simulink model "Hector"  (R2023b)
settings: Solver=daessc  StartTime=0.0  StopTime=1  FixedStep=0.001  MaxStep=1e-3  RelTol=1e-2
model workspace (MATLAB code in the model file):
  | %% World Plane
  | plane_x = 20;
  | plane_y = 2;
  | plane_z = 0.05;
  | 
  | %% motor
  | %A1
  | motor_com = [0, -0.02,0];
  | motor_com_mirror = [0, 0.02,0];
  | 
  | motor_I = [0.00048,0.00071,0.00048];
  | motor_mass = 0.605;
  | 
  | %% Body
  | % Inertial
  | body_com_x = 0.0;
  | body_com_y = 0.0;
  | body_com_z = -0.0;
  | body_mass = 5.75;
  | body_ixx = 44350*1e-6;
  | body_ixy = 0.0;
  | body_ixz = 0.0;
  | body_iyy = 53149*1e-6;
  | body_iyz = 0.0;
  | body_izz = 21390*1e-6;
  | 
  | %% Hip 1
  | % joint
  | hip1_offset_x =0.0;
  | hip1_offset_y = 0.047;
  | hip1_offset_z = 0.1265;
  | % hip1_max = 15;
  | % hip1_min = -15;
  | hip1_velocity_max = 21;
  | hip1_torque_max = 33.5;
  | % Inertial
  | hip1_com_x = 0.0268;
  | hip1_com_y = -0.00315;
  | hip1_com_z = -0.0272;
  | hip1_mass = 0.173;
  | hip1_ixx = 0.00022;
  | hip1_ixy = 0.0;
  | hip1_ixz = 0.0;
  | hip1_iyy = 0.00024;
  | hip1_iyz = 0.0;
  | hip1_izz = 0.00016;
  | 
  | %% Hip 2
  | % joint
  | hip2_offset_x =0.053;
  | hip2_offset_y = 0.0185;
  | hip2_offset_z = 0.071;
  | % hip2_max = 15;
  | % hip2_min = -15;
  | hip2_velocity_max = 21;
  | hip2_torque_max = 33.5;
  | % Inertial
  | hip2_com_x = -0.0308;
  | hip2_com_y = -0.00942;
  | hip2_com_z = 0.0;
  | hip2_mass = 0.0722;
  | hip2_ixx = 0.0000422;
  | hip2_ixy = 0.0;
  | hip2_ixz = 0.0;
  | hip2_iyy = 0.000120;
  | hip2_iyz = 0.0;
  | hip2_izz = 0.0000708;
  | 
  | %% Thigh
  | % joint
  | thigh_offset_x =-0.06;
  | thigh_offset_y = 0.004;
  | thigh_offset_z = 0.0;
  | % thigh_max = 130;
  | % thigh_min = -45;
  | thigh_velocity_max = 21;
  | thigh_torque_max = 33.5;
  | % Inertial
  | thigh_com_x = -0.00143;
  | thigh_com_y = -0.02106;
  | thigh_com_z = -0.06115;
  | thigh_mass = 0.397;
  | thigh_ixx = 0.00197;
  | thigh_ixy = 0.0;
  | thigh_ixz = 0.0;
  | thigh_iyy = 0.00218;
  | thigh_iyz = 0.0;
  | thigh_izz = 0.00033;
  | 
  | ankle_motor_offset_x = 0;
  | ankle_motor_offset_y = 0.039;
  | ankle_motor_offset_z = 0;
  | 
  | knee_motor_offset_x = 0;
  | knee_motor_offset_y = 0.039;
  | knee_motor_offset_z = -0.095;
  | 
  | %% Calf
  | % joint
  | calf_offset_x = 0.0;
  | calf_offset_y = 0.003;
  | calf_offset_z = -0.22;
  | % calf_max = 0;
  | % calf_min = -135;
  | % knee_max = 0;
  | % knee_min = -160;
  | calf_velocity_max = 14*1.5;
  | calf_torque_max = 51;
  | % Inertial
  | calf_com_x = 0.00165;
  | calf_com_y = -0.01117;
  | calf_com_z = -0.06438;
  | calf_mass = 0.136;
  | calf_ixx = 0.00071;
  | calf_ixy = 0.0;
  | calf_ixz = 0.0;
  | calf_iyy = 0.00072;
  | calf_iyz = 0.0;
  | calf_izz = 0.00002;
  | 
  | %% Toe
  | % joint
  | toe_offset_x = 0.0;
  | toe_offset_y = 0.011;
  | toe_offset_z = -0.22;
  | % toe_max = 60;
  | % toe_min = -60;
  | toe_velocity_max = 21;
  | toe_torque_max = 33.5;
  | % Inertial
  | toe_com_x = 0.00239;
  | toe_com_y = 0.00002;
  | toe_com_z = -0.02261;
  | toe_mass = 0.08425;
  | toe_ixx = 0.00001;
  | toe_ixy = 0.0;
  | toe_ixz = 0.0;
  | toe_iyy = 0.00011;
  | toe_iyz = 0.0;
  | toe_izz = 0.00011;
  | %% Contact
  | contact_front = 0.091;
  | contact_rear = -0.061;
  | contact_right = 0.026;
  | contact_left = 0.01;
  | contact_z = 0.039;
  | 
  | %%
  | %dorito
  | dorito_offset_x = 0;
  | dorito_offset_y = 0.012;
  | dorito_offset_z = 0;
  | 
  | dorito_lower_connection = [0.034 0 -0.044];
  | dorito_upper_connection = [0.034 0 0.021];
  | 
  | linkage_mass = 0.051;
  | linkage_com = [0 0 -0.11];
  | linkage_I = [0.00001 0.00002 0.00002];
  | %% Arms
  | shoulder_com_x = 0;
  | shoulder_com_y = 0;
  | shoulder_com_z = 0;
  | shoulder_mass = 0.835;
  | % shoulder_mass = 0.05;
  | shoulder_ixx = 920*1e-6;
  | shoulder_ixy = 0.0;
  | shoulder_ixz = 0.0;
  | shoulder_iyy = 270*1e-6;
  | shoulder_iyz = 0.0;
  | shoulder_izz = 499*1e-6;
  | 
  | upperarm_com_x = 0;
  | upperarm_com_y = 0;
  | upperarm_com_z = 0;
  | upperarm_mass = 1.35;
  | % upperarm_mass = 0.05;
  | upperarm_ixx = 1200*1e-6;
  | upperarm_ixy = 0.0;
  | upperarm_ixz = 0.0;
  | upperarm_iyy = 1170*1e-6;
  | upperarm_iyz = 0.0;
  | upperarm_izz = 729*1e-6;
  | 
  | forearm_com_x = 0;
  | forearm_com_y = 0;
  | forearm_com_z = -0.10;
  | forearm_mass = 0.53;
  | % forearm_mass = 0.03;
  | forearm_ixx = 427*1e-6;
  | forearm_ixy = 0.0;
  | forearm_ixz = 0.0;
  | forearm_iyy = 466*1e-6;
  | forearm_iyz = 0.0;
  | forearm_izz = 72*1e-6;
values from neighbouring files (symbols this model uses):
  body_v0 = [0 0 0]    [Initiate_Simulation.m]
  body_z0 = 0.55    [Initiate_Simulation.m]
  dt_MPC = gaitcycle/10    (= 0.04)    [Initiate_Simulation.m]
  N = 5000    [Initiate_Simulation.m]
  shoulderx_max = 90    [Initiate_Simulation.m]
  shoulderx_min = -15    [Initiate_Simulation.m]
  shoulderx_q0 = 0    [Initiate_Simulation.m]
undefined symbols (not defined in the file or in its folder): AssignMPCStage, sigbuilder_block, X, Y, Z
libraries: sm_lib x169, nesl_utility x95, dspindex x1, simulink x1
(part 1 of 7)
settings Model: Creator=alber  LastModifiedBy=chuon
settings SolverCC: DaesscMode=Balanced  ShapePreserveControl=EnableAll  ZeroCrossAlgorithm=Adaptive  AlgebraicLoopSolver=TrustRegion
settings DataIOCC: LimitDataPoints=on  MaxDataPoints=10000
settings OptimizationCC: LifeSpan=inf
settings DebuggingCC: IgnoredZcDiagnostic=none  UnconnectedInputMsg=warning  UnconnectedOutputMsg=warning  UnconnectedLineMsg=warning  AllowSymbolicDim=off  SFUnexpectedBacktrackingDiag=warning  SFNoUnconditionalDefaultTransitionDiag=warning  SFExecutionAtInitializationDiag=none  ArithmeticOperatorsInVariantConditions=warning
settings ModelReferenceCC: EnableRefExpFcnMdlSchedulingChecks=on
settings SFSimCC: SimUseLocalCustomCode=off  CustomCodeUndefinedFunction=UseInterfaceOnly
settings RTWCC: RTWUseLocalCustomCode=off  DLArmComputeVersion=19.05
settings CodeAppCC: StateflowObjectComments=on
settings GRTTargetCC: TargetLangStandard=C89/C90 (ANSI)
settings ConfigComp: CovMetricSettings=dw  CovSaveCumulativeToWorkspaceVar=on  CovSaveSingleToWorkspaceVar=on  CovExternalEMLEnable=off  CovSFcnEnable=off
settings SimscapeCC: SimscapeLogType=all  SimscapeLogSimulationStatistics=on  SimscapeLogDataHistory=10000
settings ExplorerConfigSet: InternalSimMechanicsExplorerSettings="<ExplorerConfiguration><canonicalview>default</canonicalview><AnimationSetting><BasePlaybackSpeed>1.0</BasePlaybackSpeed><PlaybackSpeedFactor>1.0</PlaybackSpeedFactor></AnimationSetting><TilePanel><TileInfo><Tiles Columns=\"1\" Count=\"1\" Rows=\"1\"><Column Weight=\"1\"/><Row Weight=\"1\"/><Tile Height=\"1\" Width=\"1\" X=\"0\" Y=\"0\"/></Tiles></TileInfo><SceneInfo><SceneViewer><BGColor><R>0.60000002384185791</R><G>0.60000002384185791</G><B>0.60000002384185791</B></BGColor><Camera><DoPerspective>off</DoPerspective><Position><X>4.09836314786391398</X><Y>-3.96594002614336105</Y><Z>4.23361424387727237</Z></Position><Center><X>-0.00094258239399230663</X><Y>0.133365704114546013</Y><Z>0.134308513619366465</Z></Center><Up><X>-0.408248290463863073</X><Y>0.408248290463863073</Y><Z>0.816496580927726145</Z></Up><ViewLimDist>1</ViewLimDist><YLim>0.846160332563345552</YLim><XLim>1.21706171949998887</XLim></Camera></SceneViewer></SceneInfo></TilePanel><MechEditorPanel><Cameras/><GfxPanelCameraMap/><VideoCreator><PlaybackSpeedRatio>1.0</PlaybackSpeedRatio><FrameRate>60</FrameRate><VideoFormat>Motion JPEG AVI</VideoFormat><FrameSize>[800 600]</FrameSize></VideoCreator></MechEditorPanel></ExplorerConfiguration>"

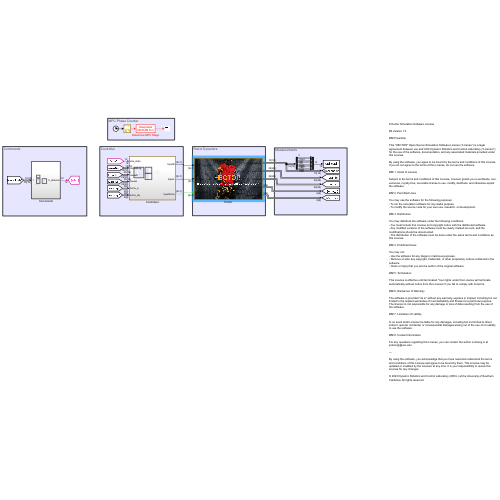
[thumbnail: Simulink's stored preview of the top-level diagram]
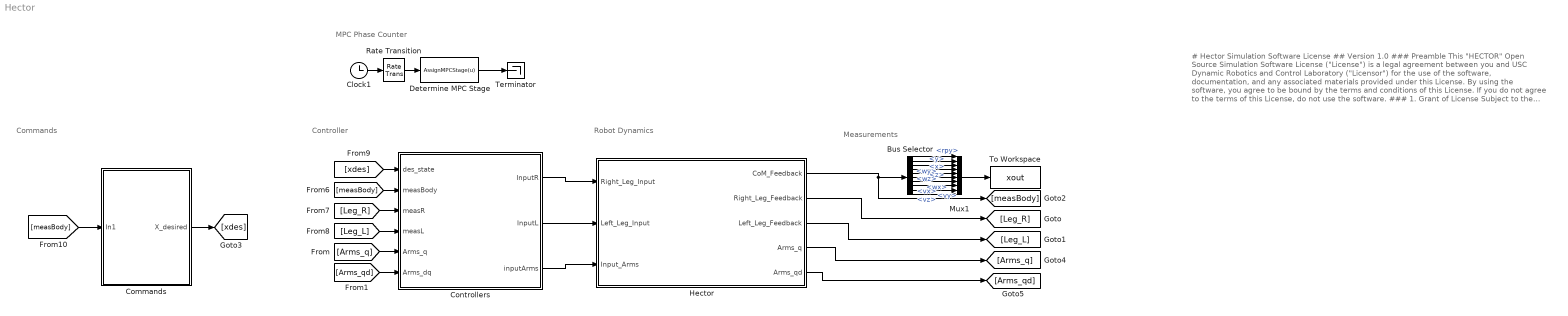
== system Hector ==
  note: # Hector Simulation Software License
      |
      | ## Version 1.0
      |
      | ### Preamble
      |
      | This "HECTOR" Open Source Simulation Software License ("License") is a legal agreement between you and USC Dynamic Robotics and Control Laboratory ("Licensor") for the use of the software, documentation, and any associated materials provided under this License.
      |
      | By using the software, you agree to be bound by the terms and conditions of this License. If you do not agree to the terms of this License, do not use the software.
      |
      | ### 1. Grant of License
      |
      | Subject to the terms and conditions of this License, Licensor grants you a worldwide, non-exclusive, royalty-free, revocable license to use, modify, distribute, and otherwise exploit the software.
      |
      | ### 2. Permitted Uses
      |
      | You may use the software for the following purposes:
      | - To run the simulation software for any lawful purpose.
      | - To modify the source code for your own use, research, or development.
      |
      | ### 3. Distribution
      |
      | You may distribute the software under the following conditions:
      | - You must include this License and copyright notice with the distributed software.
      | - Any modified versions of the software must be clearly marked as such, and the modifications should be documented.
      | - The distribution of the software must be done under the same terms and conditions as this License.
      |
      | ### 4. Prohibited Uses
      |
      | You may not:
      | - Use the software for any illegal or malicious purposes.
      | - Remove or alter any copyright, trademark, or other proprietary notices contained in the software.
      | - Claim or imply that you are the author of the original software.
      |
      | ### 5. Termination
      |
      | This License is effective until terminated. Your rights under this License will terminate automatically without notice from the Licensor if you fail to comply with its terms.
      |
      | ### 6. Disclaimer of Warranty
      |
      | The software is provided "as is" without any warranty, express or implied, including but not limited to the implied warranties of merchantability and fitness for a particular purpose. The licensor is not responsible for any damage or loss of data resulting from the use of the software.
      |
      | ### 7. Limitation of Liability
      |
      | In no event shall Licensor be liable for any damages, including but not limited to direct, indirect, special, incidental, or consequential damages arising out of the use of or inability to use the software.
      |
      | ### 8. Contact Information
      |
      | For any questions regarding this License, you can contact the author Junheng Li at junhengl@usc.edu.
      |
      | ---
      |
      | By using the software, you acknowledge that you have read and understood the terms and conditions of this License and agree to be bound by them. This License may be updated or modified by the Licensor at any time. It is your responsibility to review this License for any changes.
      |
      | © 2023 Dynamic Robotics and Control Laboratory (DRCL) at the University of Southern California. All rights reserved.
  note: Measurements
  note: MPC Phase Counter
  note: Commands
  note: Robot Dynamics
  note: Controller
  Bus Selector : BusSelector  OutputSignals=rpy,x,y,z,wz,wy,wx,vx,vy,vz
  Clock1 : Clock
  Commands : Subsystem
  Controllers : Subsystem
  Determine MPC Stage : MATLABFcn  MATLABFcn=AssignMPCStage(u)  Output1D=off
  Hector : Subsystem
      mask Display: image('$imagefile'); % Use "Edit Image" on toolstrip to change.
  Mux1 : Mux  Inputs=10
  Rate Transition : RateTransition  OutPortSampleTime=5e-4
  Terminator : Terminator
  To Workspace : ToWorkspace  VariableName=xout  SampleTime=-1
  wires:
  Hector/2(Right_Leg_Feedback) -> [Leg_R]
  Hector/3(Left_Leg_Feedback) -> [Leg_L]
  Hector/1(CoM_Feedback) -> [measBody], Bus Selector/1
  [Leg_L] -> Controllers/4(measL)
  [Leg_R] -> Controllers/3(measR)
  [measBody] -> Controllers/2(measBody)
  Controllers/1(InputR) -> Hector/1(Right_Leg_Input)
  Controllers/2(InputL) -> Hector/2(Left_Leg_Input)
  Bus Selector/1 -> Mux1/1  "<rpy>"
  Bus Selector/2 -> Mux1/2  "<x>"
  Bus Selector/3 -> Mux1/3  "<y>"
  Bus Selector/4 -> Mux1/4  "<z>"
  Bus Selector/5 -> Mux1/5  "<wz>"
  Bus Selector/7 -> Mux1/7  "<wx>"
  Bus Selector/8 -> Mux1/8  "<vx>"
  Bus Selector/9 -> Mux1/9  "<vy>"
  Bus Selector/10 -> Mux1/10  "<vz>"
  Bus Selector/6 -> Mux1/6  "<wy>"
  Mux1/1 -> To Workspace/1
  [xdes] -> Controllers/1(des_state)
  Clock1/1 -> Rate Transition/1
  Rate Transition/1 -> Determine MPC Stage/1
  [measBody] -> Commands/1(In1)
  Commands/1(X_desired) -> [xdes]
  Determine MPC Stage/1 -> Terminator/1
  Hector/4(Arms_q) -> [Arms_q]
  Hector/5(Arms_qd) -> [Arms_qd]
  Controllers/3(inputArms) -> Hector/3(Input_Arms)
  [Arms_q] -> Controllers/5(Arms_q)
  [Arms_qd] -> Controllers/6(Arms_dq)

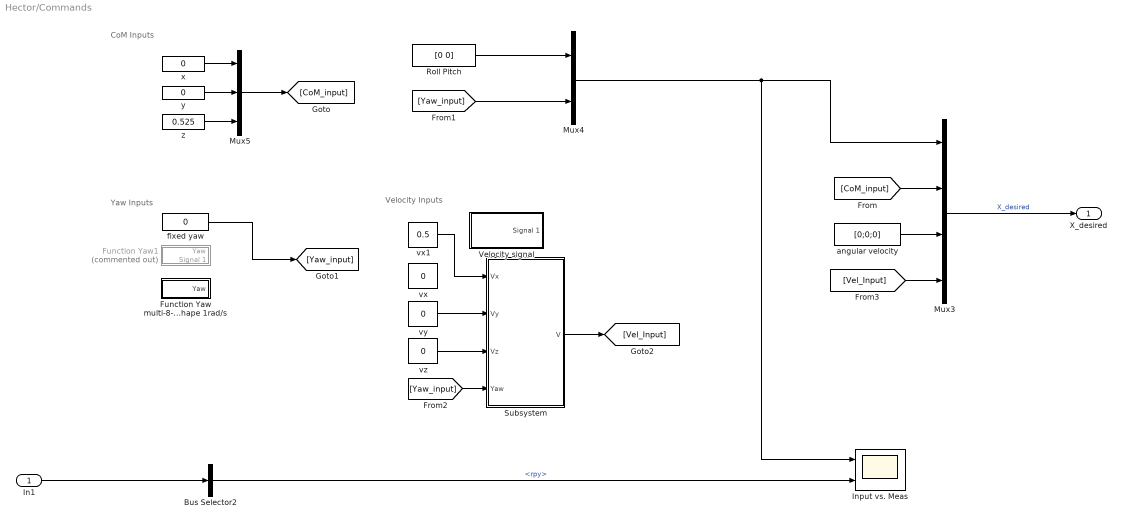
== system Hector/Commands ==
  note: Velocity Inputs
  note: CoM Inputs
  note: Yaw Inputs
  In1 : Inport
  Bus Selector2 : BusSelector  OutputSignals=rpy
  Function Yaw multi-8-shape 1rad/s : Subsystem  Tag=STV Subsys  LoadFcn=sigbuilder_block('load');  StartFcn=sigbuilder_block('start');  StopFcn=sigbuilder_block('stop');  ClipboardFcn=sigbuilder_block('clipboard');  mask(Sigbuilder block){tuvar=[0:10]}
      mask help: Simulink:masks:SigbuilderBlock_MD
      mask init:
      | if ~strcmp(get_param(bdroot(gcbh),'SimulationStatus'),'stopped') tuvar = sigbuilder_block('maskInit'); end
      settings: CopyFcn=sigbuilder_block('copy');  DeleteFcn=sigbuilder_block('delete');  ModelCloseFcn=sigbuilder_block('modelClose');  PreSaveFcn=sigbuilder_block('preSave');  PauseFcn=sigbuilder_block('pause');  ContinueFcn=sigbuilder_block('continue');  NameChangeFcn=sigbuilder_block('namechange');  OpenFcn=sigbuilder_block('open',[595.8 225 550.8 361.2 ]);  CloseFcn=sigbuilder_block('close');
      mask Display: plot(0, 0, 100, 100,[2, 2, 32, 32, 2], [68, 8, 8, 68, 68],[32, 2], [38, 38], [32, 19, 2],[53, 60, 44], [32, 17, 17, 2],[16, 16, 31, 31]);txt = getActiveGroup(gcbh);text(2, 100, txt,'verticalAlignment', 'top');
  Function Yaw1 : Subsystem  Tag=STV Subsys  Commented=on  LoadFcn=sigbuilder_block('load');  StartFcn=sigbuilder_block('start');  StopFcn=sigbuilder_block('stop');  ClipboardFcn=sigbuilder_block('clipboard');  mask(Sigbuilder block){tuvar=[0:10]}
      mask help: Simulink:masks:SigbuilderBlock_MD
      mask init:
      | if ~strcmp(get_param(bdroot(gcbh),'SimulationStatus'),'stopped') tuvar = sigbuilder_block('maskInit'); end
      settings: CopyFcn=sigbuilder_block('copy');  DeleteFcn=sigbuilder_block('delete');  ModelCloseFcn=sigbuilder_block('modelClose');  PreSaveFcn=sigbuilder_block('preSave');  PauseFcn=sigbuilder_block('pause');  ContinueFcn=sigbuilder_block('continue');  NameChangeFcn=sigbuilder_block('namechange');  OpenFcn=sigbuilder_block('open',[190.2 83.4 493.2 502.8 ]);  CloseFcn=sigbuilder_block('close');
      mask Display: plot(0, 0, 100, 100,[2, 2, 32, 32, 2], [68, 8, 8, 68, 68],[32, 2], [38, 38], [32, 19, 2],[53, 60, 44], [32, 17, 17, 2],[16, 16, 31, 31]);txt = getActiveGroup(gcbh);text(2, 100, txt,'verticalAlignment', 'top');
  Input vs. Meas : Scope  NumInputPorts=2
  Mux3 : Mux
  Mux4 : Mux  Inputs=2
  Mux5 : Mux  Inputs=3
  Roll Pitch : Constant  Value=[0 0]
  Subsystem : Subsystem
  Velocity signal : Subsystem  Tag=STV Subsys  LoadFcn=sigbuilder_block('load');  StartFcn=sigbuilder_block('start');  StopFcn=sigbuilder_block('stop');  ClipboardFcn=sigbuilder_block('clipboard');  mask(Sigbuilder block){tuvar=[0:10]}
      mask help: Simulink:masks:SigbuilderBlock_MD
      mask init:
      | if ~strcmp(get_param(bdroot(gcbh),'SimulationStatus'),'stopped') tuvar = sigbuilder_block('maskInit'); end
      settings: CopyFcn=sigbuilder_block('copy');  DeleteFcn=sigbuilder_block('delete');  ModelCloseFcn=sigbuilder_block('modelClose');  PreSaveFcn=sigbuilder_block('preSave');  PauseFcn=sigbuilder_block('pause');  ContinueFcn=sigbuilder_block('continue');  NameChangeFcn=sigbuilder_block('namechange');  OpenFcn=sigbuilder_block('open',[439.8 157.8 550.8 400.2 ]);  CloseFcn=sigbuilder_block('close');
      mask Display: plot(0, 0, 100, 100,[2, 2, 32, 32, 2], [68, 8, 8, 68, 68],[32, 2], [38, 38], [32, 19, 2],[53, 60, 44], [32, 17, 17, 2],[16, 16, 31, 31]);txt = getActiveGroup(gcbh);text(2, 100, txt,'verticalAlignment', 'top');
  angular velocity : Constant  Value=[0;0;0]
  fixed yaw : Constant  Value=0
  vx : Constant  Value=0
  vx1 : Constant  Value=0.5
  vy : Constant  Value=0
  vz : Constant  Value=0
  x : Constant  Value=0
  y : Constant  Value=0
  z : Constant  Value=0.525
  X_desired : Outport
  wires:
  y/1 -> Mux5/2
  Mux4/1 -> Mux3/1, Input vs. Meas/1
  x/1 -> Mux5/1
  angular velocity/1 -> Mux3/3
  Roll Pitch/1 -> Mux4/1
  z/1 -> Mux5/3
  In1/1 -> Bus Selector2/1
  Bus Selector2/1 -> Input vs. Meas/2  "<rpy>"
  Mux3/1 -> X_desired/1  "X_desired"
  Mux5/1 -> [CoM_input]
  [CoM_input] -> Mux3/2
  vx1/1 -> Subsystem/1(Vx)
  vy/1 -> Subsystem/2(Vy)
  vz/1 -> Subsystem/3(Vz)
  fixed yaw/1 -> [Yaw_input]
  [Yaw_input] -> Mux4/2
  [Yaw_input] -> Subsystem/4(Yaw)
  Subsystem/1(V) -> [Vel_Input]
  [Vel_Input] -> Mux3/4

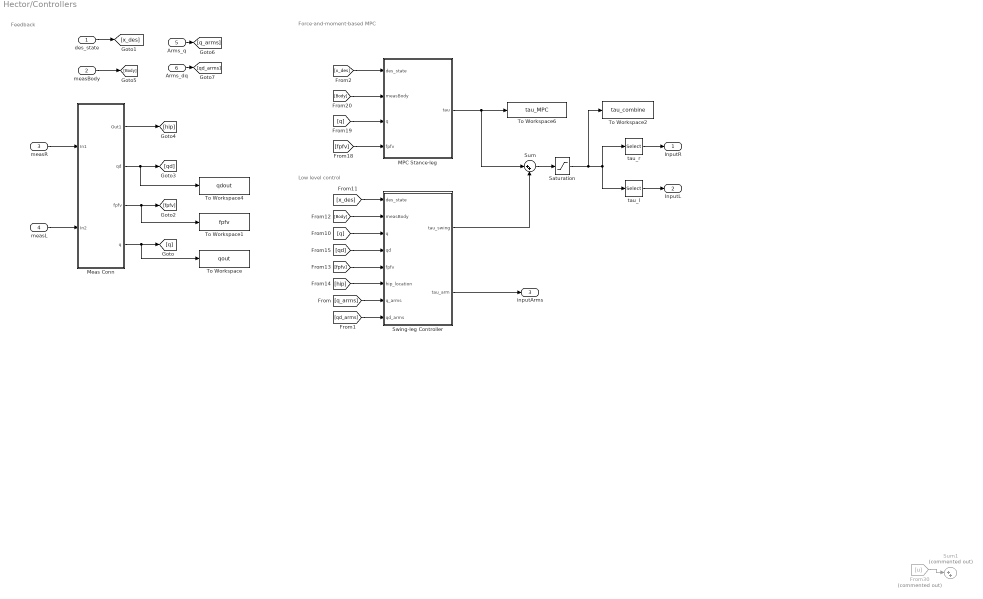
== system Hector/Controllers ==
  note: Low level control
  note: Force-and-moment-based MPC
  note: Feedback
  des_state : Inport
  measBody : Inport  Port=2
  measR : Inport  Port=3
  measL : Inport  Port=4
  Arms_q : Inport  Port=5
  Arms_dq : Inport  Port=6
  From30 : From  Commented=on  GotoTag=u
  MPC Stance-leg : Subsystem  TreatAsAtomicUnit=on
  Meas Conn : Subsystem
  Saturation : Saturate  UpperLimit=[33.5;33.5;33.5;51;33.5;33.5;33.5;33.5;51;33.5]*1  LowerLimit=-[33.5;33.5;33.5;51;33.5;33.5;33.5;33.5;51;33.5]*1
  Sum : Sum  Inputs=|++
  Sum1 : Sum  Commented=on  Inputs=|++
  "Swing-leg Controller " : Subsystem
  To Workspace : ToWorkspace  VariableName=qout  SampleTime=-1
  To Workspace1 : ToWorkspace  VariableName=fpfv  SampleTime=-1
  To Workspace2 : ToWorkspace  VariableName=tau_combine  SampleTime=-1
  To Workspace4 : ToWorkspace  VariableName=qdout  SampleTime=-1
  To Workspace6 : ToWorkspace  VariableName=tau_MPC  SampleTime=-1
  tau_l : Selector  InputPortWidth=10  IndexOptions=Index vector (dialog)  Indices=[6:10]  OutputSizes=1
  tau_r : Selector  InputPortWidth=10  IndexOptions=Index vector (dialog)  Indices=[1:5]  OutputSizes=1
  InputR : Outport
  InputL : Outport  Port=2
  inputArms : Outport  Port=3
  wires:
  measBody/1 -> [Body]
  tau_r/1 -> InputR/1
  tau_l/1 -> InputL/1
  Saturation/1 -> To Workspace2/1, tau_l/1, tau_r/1
  Sum/1 -> Saturation/1
  des_state/1 -> [x_des]
  [x_des] -> MPC Stance-leg/1(des_state)
  [x_des] -> "Swing-leg Controller "/1(des_state)
  [Body] -> "Swing-leg Controller "/2(measBody)
  [q] -> "Swing-leg Controller "/3(q)
  [fpfv] -> "Swing-leg Controller "/5(fpfv)
  [hip] -> "Swing-leg Controller "/6(hip_location)
  [qd] -> "Swing-leg Controller "/4(qd)
  From30/1 -> Sum1/1
  [Body] -> MPC Stance-leg/2(measBody)
  [fpfv] -> MPC Stance-leg/4(fpfv)
  [q] -> MPC Stance-leg/3(q)
  "Swing-leg Controller "/1(tau_swing) -> Sum/2
  MPC Stance-leg/1(tau) -> To Workspace6/1, Sum/1
  Meas Conn/3(fpfv) -> [fpfv], To Workspace1/1
  Meas Conn/4(q) -> [q], To Workspace/1
  Meas Conn/2(qd) -> [qd], To Workspace4/1
  measR/1 -> Meas Conn/1(In1)
  measL/1 -> Meas Conn/2(In2)
  Meas Conn/1(Out1) -> [hip]
  Arms_q/1 -> [q_arms]
  Arms_dq/1 -> [qd_arms]
  "Swing-leg Controller "/2(tau_arm) -> inputArms/1
  [q_arms] -> "Swing-leg Controller "/7(q_arms)
  [qd_arms] -> "Swing-leg Controller "/8(qd_arms)

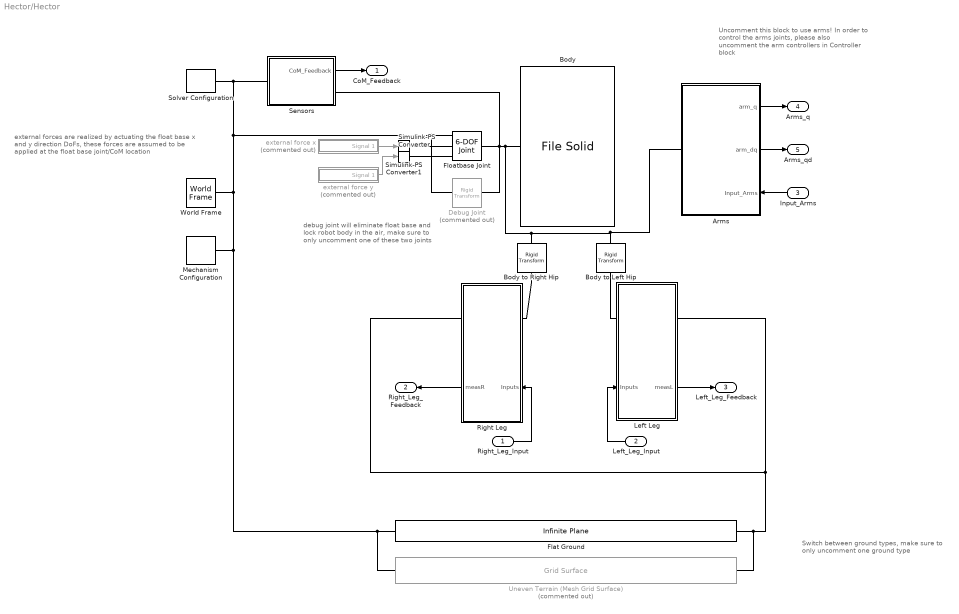
== system Hector/Hector ==
  note: external forces are realized by actuating the float base
      | x and y direction DoFs, these forces are assumed to
      | be applied at the float base joint/CoM location
  note: debug joint will eliminate float base
      | and lock robot body in the air, make
      | sure to only uncomment one of these
      | two joints
  note: Switch between ground types, make sure to
      | only uncomment one ground type
  note: Uncomment this block to use arms!
      | In order to control the arms joints,
      | please also uncomment the arm controllers
      | in Controller block
  Right_Leg_Input : Inport
  Left_Leg_Input : Inport  Port=2
  Input_Arms : Inport  Port=3
  Arms : Subsystem
      settings: PortSchema="{\"entries\":[{\"content\":{\"sides\":[{\"content\":{\"connectorIds\":[\"LConn1\"]},\"type\":\"ConnectorPlacement.EquallySpacedRectSide\",\"uuid\":\"a2f749fc-f9bc-4cf5-9bf3-19861dfd7706\"},{\"content\":{\"connectorIds\":[\"Out1\",\"Out2\",\"In1\"],\"side\":\"RIGHT\"},\"type\":\"ConnectorPlacement.EquallySpacedRectSide\",\"uuid\":\"def031a3-c275-4480-958b-61894f4750cc\"},{\"content\":{\"side\":\"TOP\"},\"type\":\"ConnectorPlacement.EquallySpacedRectSide\",\"uuid\":\"3d1c74ca-aaa2-47cb-b1e3-b44b534dece8\"},{\"content\":{\"side\":\"BOTTOM\"},\"type\":\"ConnectorPlacement.EquallySpacedRectSide\",\"uuid\":\"4dd24460-d3b9-42d8-9cbf-9842bc34e6d5\"}]},\"type\":\"ConnectorPlacement.EquallySpacedConnector\",\"uuid\":\"d1dc773b-a4cf-42cb-99a0-e241de2bfabf\"}],\"packageUris\":[\"http://schema.mathworks.com/mf0/Connector/R2020b\"],\"version\":\"1.0\"}"
  Body : sm_lib/Body Elements/File Solid  ExtGeomFileName=STL files\body.STL  UnitType=Custom  ExtGeomFileUnits=m  StepReaderType=HEX  ExportConvexHullGeometry=off  InertiaType=Custom  Mass=body_mass  MassUnits=kg  CenterOfMass=[body_com_x body_com_y body_com_z]  CenterOfMassUnits=m  MomentsOfInertia=[body_ixx body_iyy body_izz]  MomentsOfInertiaUnits=kg*m^2  ProductsOfInertia=[0 0 0]  ProductsOfInertiaUnits=kg*m^2  BasedOnType=Density  Density=1000  DensityUnits=kg/m^3  DoExposeReferenceFrame=on  SerializedFrames=<Frames/>  GraphicType=FromGeometry  MarkerShape=Sphere  MarkerSize=10  GraphicVisPropType=SimpleVisualProperties  GraphicDiffuseColor=[0.2 0.2 0.2]  GraphicSpecularColor=[0.2 0.2 0.2 1.0]  GraphicAmbientColor=[0.25 0.25 0.25 1.0]  GraphicEmissiveColor=[0.0 0.0 0.0 1.0]  GraphicShininess=8  GraphicOpacity=0.9
  Body to Left Hip : sm_lib/Frames and Transforms/Rigid Transform  TranslationMethod=Cartesian  TranslationStandardOffset=0  TranslationStandardOffsetUnits=m  TranslationStandardAxis=+Z  TranslationCartesianOffset="[hip1_offset_x  hip1_offset_y -hip1_offset_z]"  TranslationCartesianOffsetUnits=m  TranslationROffset=0  TranslationROffsetUnits=m  TranslationZOffset=0  TranslationZOffsetUnits=m  TranslationThetaOffset=0  TranslationThetaOffsetUnits=deg  RotationMethod=None  RotationAngleUnits=deg  RotationStandardAxis=+Z  RotationAngle=0.0  RotationArbitraryAxis=[0 0 1]  FollAlignAxisA=+X  BaseAlignAxisA=+Y  FollAlignAxisB=+Y  BaseAlignAxisB=+Z  RotationSequenceAxes=FollowerAxes  RotationSequence=XYX  RotationSequenceAngles=[0 0 0]  RotationSequenceAnglesUnits=deg  RotationMatrix=[1 0 0; 0 1 0; 0 0 1]  Quaternion=[1 0 0 0]
  Body to Right Hip : sm_lib/Frames and Transforms/Rigid Transform  TranslationMethod=Cartesian  TranslationStandardOffset=0  TranslationStandardOffsetUnits=m  TranslationStandardAxis=+Z  TranslationCartesianOffset="[hip1_offset_x  -hip1_offset_y -hip1_offset_z]"  TranslationCartesianOffsetUnits=m  TranslationROffset=0  TranslationROffsetUnits=m  TranslationZOffset=0  TranslationZOffsetUnits=m  TranslationThetaOffset=0  TranslationThetaOffsetUnits=deg  RotationMethod=None  RotationAngleUnits=deg  RotationStandardAxis=+Z  RotationAngle=0.0  RotationArbitraryAxis=[0 0 1]  FollAlignAxisA=+X  BaseAlignAxisA=+Y  FollAlignAxisB=+Y  BaseAlignAxisB=+Z  RotationSequenceAxes=FollowerAxes  RotationSequence=XYX  RotationSequenceAngles=[0 0 0]  RotationSequenceAnglesUnits=deg  RotationMatrix=[1 0 0; 0 1 0; 0 0 1]  Quaternion=[1 0 0 0]
  Debug Joint : sm_lib/Frames and Transforms/Rigid Transform  Commented=on  TranslationMethod=Cartesian  TranslationStandardOffset=0  TranslationStandardOffsetUnits=m  TranslationStandardAxis=+Z  TranslationCartesianOffset=[0 0 body_z0+0.1]  TranslationCartesianOffsetUnits=m  TranslationROffset=0  TranslationROffsetUnits=m  TranslationZOffset=0  TranslationZOffsetUnits=m  TranslationThetaOffset=0  TranslationThetaOffsetUnits=deg  RotationMethod=None  RotationAngleUnits=deg  RotationStandardAxis=+Z  RotationAngle=0.0  RotationArbitraryAxis=[0 0 1]  FollAlignAxisA=+X  BaseAlignAxisA=+Y  FollAlignAxisB=+Y  BaseAlignAxisB=+Z  RotationSequenceAxes=FollowerAxes  RotationSequence=XYX  RotationSequenceAngles=[0 0 0]  RotationSequenceAnglesUnits=deg  RotationMatrix=[1 0 0; 0 1 0; 0 0 1]  Quaternion=[1 0 0 0]
  Flat Ground : sm_lib/Curves and Surfaces/Infinite Plane  GraphicType=Rectangle  GraphicPlaneWidth=10  GraphicPlaneWidthUnits=m  GraphicPlaneHeight=10  GraphicPlaneHeightUnits=m  GraphicVisPropType=SimpleVisualProperties  GraphicDiffuseColor=[0.5 0.75 0.5]  GraphicOpacity=0.75  GraphicSpecularColor=[0.5 0.5 0.5 1.0]  GraphicAmbientColor=[0.15 0.15 0.15 1.0]  GraphicEmissiveColor=[0.0 0.0 0.0 1.0]  GraphicShininess=75
  Floatbase Joint : sm_lib/Joints/6-DOF Joint  JointMode=Normal  SenseConstraintForce=off  SenseConstraintForceX=off  SenseConstraintForceY=off  SenseConstraintForceZ=off  SenseConstraintTorque=off  SenseConstraintTorqueX=off  SenseConstraintTorqueY=off  SenseConstraintTorqueZ=off  SenseTotalForce=off  SenseTotalForceX=off  SenseTotalForceY=off  SenseTotalForceZ=off  SenseTotalTorque=off  SenseTotalTorqueX=off  SenseTotalTorqueY=off  SenseTotalTorqueZ=off  CompositeWrenchDir=FollowerOnBase  CompositeWrenchFrame=BaseFrame  PxEquilibriumPosition=0  PxEquilibriumPositionUnits=m  PxSpringStiffness=0  PxSpringStiffnessUnits=N/m  PxDampingCoefficient=world_damping  PxDampingCoefficientUnits=N/(m/s)  PxTorqueActuationMode=InputTorque  PxMotionActuationMode=ComputedMotion  PxSensePosition=off  PxSenseVelocity=off  PxSenseAcceleration=off  PxSenseTorqueForce=off  PxSenseLowerLimitTorqueForce=off  PxSenseUpperLimitTorqueForce=off  PxLowerLimitSpecify=off  PxLowerLimitBound=-1  PxLowerLimitBoundUnits=m  PxLowerLimitStiffness=1e6  PxLowerLimitStiffnessUnits=N/m  PxLowerLimitDamping=1e3  PxLowerLimitDampingUnits=N/(m/s)  PxLowerLimitTransitionRegionWidth=1e-4  PxLowerLimitTransitionRegionWidthUnits=m  PxUpperLimitSpecify=off  PxUpperLimitBound=1  PxUpperLimitBoundUnits=m  PxUpperLimitStiffness=1e6  PxUpperLimitStiffnessUnits=N/m  PxUpperLimitDamping=1e3  PxUpperLimitDampingUnits=N/(m/s)  PxUpperLimitTransitionRegionWidth=1e-4  PxUpperLimitTransitionRegionWidthUnits=m  PxPositionTargetSpecify=on  PxPositionTargetPriority=High  PxPositionTargetValue=body_x0  PxPositionTargetValueUnits=m  PxVelocityTargetSpecify=on  PxVelocityTargetPriority=High  PxVelocityTargetValue=body_v0(1)  PxVelocityTargetValueUnits=m/s  PyEquilibriumPosition=0  PyEquilibriumPositionUnits=m  PySpringStiffness=0  PySpringStiffnessUnits=N/m  PyDampingCoefficient=world_damping  PyDampingCoefficientUnits=N/(m/s)  PyTorqueActuationMode=InputTorque  PyMotionActuationMode=ComputedMotion  PySensePosition=off  PySenseVelocity=off  PySenseAcceleration=off  PySenseTorqueForce=off  PySenseLowerLimitTorqueForce=off  PySenseUpperLimitTorqueForce=off  PyLowerLimitSpecify=off  PyLowerLimitBound=-1  PyLowerLimitBoundUnits=m  PyLowerLimitStiffness=1e6  PyLowerLimitStiffnessUnits=N/m  PyLowerLimitDamping=1e3  PyLowerLimitDampingUnits=N/(m/s)  PyLowerLimitTransitionRegionWidth=1e-4  PyLowerLimitTransitionRegionWidthUnits=m  PyUpperLimitSpecify=off  PyUpperLimitBound=1  PyUpperLimitBoundUnits=m  PyUpperLimitStiffness=1e6  PyUpperLimitStiffnessUnits=N/m  PyUpperLimitDamping=1e3  PyUpperLimitDampingUnits=N/(m/s)  PyUpperLimitTransitionRegionWidth=1e-4  PyUpperLimitTransitionRegionWidthUnits=m  PyPositionTargetSpecify=on  PyPositionTargetPriority=High  PyPositionTargetValue=body_y0  PyPositionTargetValueUnits=m  PyVelocityTargetSpecify=on  PyVelocityTargetPriority=High  PyVelocityTargetValue=body_v0(2)  PyVelocityTargetValueUnits=m/s  PzEquilibriumPosition=0  PzEquilibriumPositionUnits=m  PzSpringStiffness=0  PzSpringStiffnessUnits=N/m  PzDampingCoefficient=world_damping  PzDampingCoefficientUnits=N/(m/s)  PzTorqueActuationMode=NoTorque  PzMotionActuationMode=ComputedMotion  PzSensePosition=off  PzSenseVelocity=off  PzSenseAcceleration=off  PzSenseTorqueForce=off  PzSenseLowerLimitTorqueForce=off  PzSenseUpperLimitTorqueForce=off  PzLowerLimitSpecify=off  PzLowerLimitBound=-1  PzLowerLimitBoundUnits=m  PzLowerLimitStiffness=1e6  PzLowerLimitStiffnessUnits=N/m  PzLowerLimitDamping=1e3  PzLowerLimitDampingUnits=N/(m/s)  PzLowerLimitTransitionRegionWidth=1e-4  PzLowerLimitTransitionRegionWidthUnits=m  PzUpperLimitSpecify=off  PzUpperLimitBound=1  PzUpperLimitBoundUnits=m  PzUpperLimitStiffness=1e6  PzUpperLimitStiffnessUnits=N/m  PzUpperLimitDamping=1e3  PzUpperLimitDampingUnits=N/(m/s)  PzUpperLimitTransitionRegionWidth=1e-4  PzUpperLimitTransitionRegionWidthUnits=m  PzPositionTargetSpecify=on  PzPositionTargetPriority=High  PzPositionTargetValue=body_z0  PzPositionTargetValueUnits=m  PzVelocityTargetSpecify=off  PzVelocityTargetPriority=High  PzVelocityTargetValue=0  PzVelocityTargetValueUnits=m/s  SphEqPosRotationMethod=None  SphEqPosRotationAngleUnits=deg  SphEqPosRotationStandardAxis=+Z  SphEqPosRotationAngle=0.0  SphEqPosRotationArbitraryAxis=[0 0 1]  SphEqPosFollAlignAxisA=+X  SphEqPosBaseAlignAxisA=+Y  SphEqPosFollAlignAxisB=+Y  SphEqPosBaseAlignAxisB=+Z  SphEqPosRotationSequenceAxes=FollowerAxes  SphEqPosRotationSequence=XYX  SphEqPosRotationSequenceAngles=[0 0 0]  SphEqPosRotationSequenceAnglesUnits=deg  SphEqPosRotationMatrix=[1 0 0; 0 1 0; 0 0 1]  SphEqPosQuaternion=[1 0 0 0]  SphSpringStiffness=0  SphSpringStiffnessUnits=N*m/deg  SphDampingCoefficient=world_rot_damping  SphDampingCoefficientUnits=N*m/(rad/s)  SphActuateTorqueX=off  SphActuateTorqueY=off  SphActuateTorqueZ=off  SphActuateTorque=off  SphTorqueActuationMode=NoTorque  SphMotionActuationMode=ComputedMotion  SphActuationFrame=BaseFrame  SphSensePosition=off  SphSenseVelocityX=off  SphSenseVelocityY=off  SphSenseVelocityZ=off  SphSenseVelocity=off  SphSenseAccelerationX=off  SphSenseAccelerationY=off  SphSenseAccelerationZ=off  SphSenseAcceleration=off  SphSenseTorqueX=off  SphSenseTorqueY=off  SphSenseTorqueZ=off  SphSenseTorqueForce=off  SphSenseLowerLimitTorqueMag=off  SphSenseUpperLimitTorqueMag=off  SphSensingFrame=BaseFrame  SphLowerLimitSpecify=off  SphLowerLimitBound=15  SphLowerLimitBoundUnits=deg  SphLowerLimitStiffness=1e4  SphLowerLimitStiffnessUnits=N*m/deg  SphLowerLimitDamping=10  SphLowerLimitDampingUnits=N*m/(deg/s)  SphLowerLimitTransitionRegionWidth=0.1  SphLowerLimitTransitionRegionWidthUnits=deg  SphUpperLimitSpecify=off  SphUpperLimitBound=45  SphUpperLimitBoundUnits=deg  SphUpperLimitStiffness=1e4  SphUpperLimitStiffnessUnits=N*m/deg  SphUpperLimitDamping=10  SphUpperLimitDampingUnits=N*m/(deg/s)  SphUpperLimitTransitionRegionWidth=0.1  SphUpperLimitTransitionRegionWidthUnits=deg  SphPositionTargetRotationMethod=RotationSequence  SphPositionTargetRotationAngleUnits=deg  SphPositionTargetRotationStandardAxis=+Y  SphPositionTargetRotationAngle=10  SphPositionTargetRotationArbitraryAxis=[0 0 1]  SphPositionTargetFollAlignAxisA=+X  SphPositionTargetBaseAlignAxisA=+Y  SphPositionTargetFollAlignAxisB=+Y  SphPositionTargetBaseAlignAxisB=+Z  SphPositionTargetRotationSequenceAxes=BaseAxes  SphPositionTargetRotationSequence=XYZ  SphPositionTargetRotationSequenceAngles=body_R  SphPositionTargetRotationSequenceAnglesUnits=deg  SphPositionTargetRotationMatrix=[1 0 0; 0 1 0; 0 0 1]  SphPositionTargetQuaternion=[1 0 0 0]  SphPositionTargetSpecify=on  SphPositionTargetPriority=High  SphVelocityTargetValue=[0 0 0]  SphVelocityTargetValueUnits=deg/s  SphVelocityTargetSpecify=off  SphVelocityTargetPriority=High  SphVelocityTargetInFollowerFrame=on
  Left Leg : Subsystem
      settings: PortSchema="{\"entries\":[{\"content\":{\"sides\":[{\"content\":{\"connectorIds\":[\"LConn1\",\"In1\"]},\"type\":\"ConnectorPlacement.EquallySpacedRectSide\",\"uuid\":\"90659dc0-2afc-4798-b2db-3c1150d3a4bf\"},{\"content\":{\"connectorIds\":[\"RConn1\",\"Out1\"],\"side\":\"RIGHT\"},\"type\":\"ConnectorPlacement.EquallySpacedRectSide\",\"uuid\":\"c522685b-3dfb-475b-9099-fd4cb10408ff\"},{\"content\":{\"side\":\"TOP\"},\"type\":\"ConnectorPlacement.EquallySpacedRectSide\",\"uuid\":\"4d7b3b8c-656f-47d5-92ce-682631add928\"}]},\"type\":\"ConnectorPlacement.EquallySpacedConnector\",\"uuid\":\"b378d38c-e18d-4cad-9e9d-e1c5ed2f56ff\"}],\"packageUris\":[\"http://schema.mathworks.com/mf0/Connector/R2020b\"],\"version\":\"1.0\"}"
  Mechanism Configuration : sm_lib/Utilities/Mechanism Configuration  UniformGravity=Constant  GravityVector=[0 0 -9.80665]  GravityVectorUnits=m/s^2  LinearizationDelta=0.001  JointModeTransitionNonlinearIterations=2
  Right Leg : Subsystem
      settings: PortSchema="{\"entries\":[{\"content\":{\"sides\":[{\"content\":{\"connectorIds\":[\"LConn1\",\"In1\"]},\"type\":\"ConnectorPlacement.EquallySpacedRectSide\",\"uuid\":\"4f14ed36-5226-4e72-a630-1f8daa80b429\"},{\"content\":{\"connectorIds\":[\"RConn1\",\"Out1\"],\"side\":\"RIGHT\"},\"type\":\"ConnectorPlacement.EquallySpacedRectSide\",\"uuid\":\"b2e3fd67-f205-455c-b895-13f2383c0153\"},{\"content\":{\"side\":\"TOP\"},\"type\":\"ConnectorPlacement.EquallySpacedRectSide\",\"uuid\":\"bfa362dd-5ada-43c1-8968-0928634d8c97\"}]},\"type\":\"ConnectorPlacement.EquallySpacedConnector\",\"uuid\":\"923760f4-20a3-4169-965c-c30ad1b161c9\"}],\"packageUris\":[\"http://schema.mathworks.com/mf0/Connector/R2020b\"],\"version\":\"1.0\"}"
  Sensors : Subsystem
  Simulink-PS Converter : nesl_utility/Simulink-PS Converter  PhysicalDomain=network_engine_domain  SubClassName=ps_input  LeftPortType=input  RightPortType=output  PseudoPeriodic=off  Frequencies=[]  NoiseDistribution=none  NoiseParameters=[]  Unit=1  AffineConversion=off  FilteringAndDerivatives=provide  SimscapeFilterOrder=1  InputFilterTimeConstant=0.001  UdotUserProvided=0
  Simulink-PS Converter1 : nesl_utility/Simulink-PS Converter  PhysicalDomain=network_engine_domain  SubClassName=ps_input  LeftPortType=input  RightPortType=output  PseudoPeriodic=off  Frequencies=[]  NoiseDistribution=none  NoiseParameters=[]  Unit=1  AffineConversion=off  FilteringAndDerivatives=provide  SimscapeFilterOrder=1  InputFilterTimeConstant=0.001  UdotUserProvided=0
  Solver Configuration : nesl_utility/Solver Configuration  PhysicalDomain=network_engine_domain  SubClassName=solver  LeftPortType=input  RightPortType=generic  Tones=[]  Harmonics=[]  SimulateNoise=off  Profile=off  UseLocalSampling=off  EnableSwitchedLinearOptims=on  FrequencyDomain=off  UseCCode=off  RelTol=0.001  AbsTol=1e-06  MinStep=1e-09  ToWorkspace=off  RevertToSquareIcSolve=off  NumHomotopyIterations=100  PhasorMode=off  PhasorModeNumHarmonics=1  ConsistencySolver=NEWTON_FTOL  IndexReductionMethod=DerivativeReplacement  DoDC=off  ResidualTolerance=1e-09  ConsistencyTolSource=GLOBAL  ConsistencyAbsTol=0.001  ConsistencyRelTol=0.001  ConsistencyTolFactor=0.001  UseLocalSolver=off  LocalSolverChoice=NE_BACKWARD_EULER_ADVANCER  ResolveIndetEquations=on  FunctionEvalNumThread=1  LocalSolverSampleTime=0.001  DoFixedCost=off  MaxNonlinIter=3  MaxModeIter=2  ComputeImpulses=off  ImpulseIterations=2  LinearAlgebra=Sparse  LinearAlgebraNumThread=0  EquationFormulation=NE_TIME_EF  DelaysMemoryBudget=1024  AutomaticFiltering=on  FilteringTimeConstant=0.001  PartitionStorageMethod=AS_NEEDED  PartitionMemoryBudget=1024  PartitionMethod=FAST  MultibodyUseLocalSolver=off  MultibodyLocalSolverChoice=ODE1  MultibodyLocalSolverSampleTime=0.001
  Uneven Terrain (Mesh Grid Surface) : sm_lib/Curves and Surfaces/Grid Surface  Commented=on  XGridVector=x_grid  XGridVectorUnits=m  YGridVector=y_grid  YGridVectorUnits=m  ZHeights=z_heights  ZHeightsUnits=m  GraphicType=FromGeometry  GraphicVisPropType=SimpleVisualProperties  GraphicDiffuseColor=[0.6745 0.9882 0.6745]  GraphicOpacity=1.0  GraphicSpecularColor=[0.5 0.5 0.5 1.0]  GraphicAmbientColor=[0.15 0.15 0.15 1.0]  GraphicEmissiveColor=[0.0 0.0 0.0 1.0]  GraphicShininess=75
  World Frame : sm_lib/Frames and Transforms/World Frame
  external force x : Subsystem  Tag=STV Subsys  Commented=on  LoadFcn=sigbuilder_block('load');  StartFcn=sigbuilder_block('start');  StopFcn=sigbuilder_block('stop');  ClipboardFcn=sigbuilder_block('clipboard');  mask(Sigbuilder block){tuvar=[0:10]}
      mask help: Simulink:masks:SigbuilderBlock_MD
      mask init:
      | if ~strcmp(get_param(bdroot(gcbh),'SimulationStatus'),'stopped') tuvar = sigbuilder_block('maskInit'); end
      settings: CopyFcn=sigbuilder_block('copy');  DeleteFcn=sigbuilder_block('delete');  ModelCloseFcn=sigbuilder_block('modelClose');  PreSaveFcn=sigbuilder_block('preSave');  PauseFcn=sigbuilder_block('pause');  ContinueFcn=sigbuilder_block('continue');  NameChangeFcn=sigbuilder_block('namechange');  OpenFcn=sigbuilder_block('open',[437.6 199.2 550.4 400 ]);  CloseFcn=sigbuilder_block('close');
      mask Display: plot(0, 0, 100, 100,[2, 2, 32, 32, 2], [68, 8, 8, 68, 68],[32, 2], [38, 38], [32, 19, 2],[53, 60, 44], [32, 17, 17, 2],[16, 16, 31, 31]);txt = getActiveGroup(gcbh);text(2, 100, txt,'verticalAlignment', 'top');
  external force y : Subsystem  Tag=STV Subsys  Commented=on  LoadFcn=sigbuilder_block('load');  StartFcn=sigbuilder_block('start');  StopFcn=sigbuilder_block('stop');  ClipboardFcn=sigbuilder_block('clipboard');  mask(Sigbuilder block){tuvar=[0:10]}
      mask help: Simulink:masks:SigbuilderBlock_MD
      mask init:
      | if ~strcmp(get_param(bdroot(gcbh),'SimulationStatus'),'stopped') tuvar = sigbuilder_block('maskInit'); end
      settings: CopyFcn=sigbuilder_block('copy');  DeleteFcn=sigbuilder_block('delete');  ModelCloseFcn=sigbuilder_block('modelClose');  PreSaveFcn=sigbuilder_block('preSave');  PauseFcn=sigbuilder_block('pause');  ContinueFcn=sigbuilder_block('continue');  NameChangeFcn=sigbuilder_block('namechange');  OpenFcn=sigbuilder_block('open',[437.6 199.2 550.4 400 ]);  CloseFcn=sigbuilder_block('close');
      mask Display: plot(0, 0, 100, 100,[2, 2, 32, 32, 2], [68, 8, 8, 68, 68],[32, 2], [38, 38], [32, 19, 2],[53, 60, 44], [32, 17, 17, 2],[16, 16, 31, 31]);txt = getActiveGroup(gcbh);text(2, 100, txt,'verticalAlignment', 'top');
  CoM_Feedback : Outport
  Right_Leg_Feedback : Outport  Port=2
  Left_Leg_Feedback : Outport  Port=3
  Arms_q : Outport  Port=4
  Arms_qd : Outport  Port=5
  wires:
  Right Leg/1(measR) -> Right_Leg_Feedback/1
  Left Leg/1(measL) -> Left_Leg_Feedback/1
  Right_Leg_Input/1 -> Right Leg/1(Inputs)
  Left_Leg_Input/1 -> Left Leg/1(Inputs)
  Sensors/1(CoM_Feedback) -> CoM_Feedback/1
  external force x/1(Signal 1) -> Simulink-PS Converter1/1
  external force y/1(Signal 1) -> Simulink-PS Converter/1
  Arms/2(arm_dq) -> Arms_qd/1
  Arms/1(arm_q) -> Arms_q/1
  Input_Arms/1 -> Arms/1(Input_Arms)
  connections:
  Body/RConn1 -- Debug Joint/RConn1 -- Sensors/RConn1 -- Floatbase Joint/RConn1 -- Arms/LConn1 -- Body to Left Hip/LConn1 -- Body to Right Hip/LConn1
  World Frame/RConn1 -- Uneven Terrain (Mesh Grid Surface)/LConn1 -- Flat Ground/LConn1 -- Mechanism Configuration/RConn1 -- Debug Joint/LConn1 -- Floatbase Joint/LConn1 -- Solver Configuration/RConn1 -- Sensors/LConn1
  Body to Right Hip/RConn1 -- Right Leg/LConn1
  Body to Left Hip/RConn1 -- Left Leg/LConn1
  Uneven Terrain (Mesh Grid Surface)/RConn1 -- Flat Ground/RConn1 -- Right Leg/RConn1 -- Left Leg/RConn1
  Simulink-PS Converter1/RConn1 -- Floatbase Joint/LConn2
  Simulink-PS Converter/RConn1 -- Floatbase Joint/LConn3

== system Hector/Commands/Function Yaw multi-8-shape 1rad//s ==
  Demux : Demux  Tag=STV Demux  Outputs=1
      settings: DisplayOption=none
  FromWs : FromWorkspace  Tag=STV FromWs  VariableName=tuvar
      SigBuilderData=|
      | common.afterFinalStr = 'Extrapolate'
      | common.sampleTime = 0
      | dataSet.timeRange = [0 50]
      | dataSet.name = 'Group 1'
      | sbobj.Groups.Name = 'Group 1'
      | sbobj.Groups.Signals.Name = 'Yaw'
      | sbobj.Groups.Signals.XData = [0 3 9 15 21 24 50]
      | sbobj.Groups.Signals.YData = [0 2 -2 2 -2 0 0]
      | sbobj.Groups.TimeRange = [0 50]
  Yaw : Outport  Tag=STV Outport
  wires:
  FromWs/1 -> Demux/1
  Demux/1 -> Yaw/1

== system Hector/Commands/Function Yaw1 ==
  Demux : Demux  Tag=STV Demux  Outputs=2
      settings: DisplayOption=none
  FromWs : FromWorkspace  Tag=STV FromWs  VariableName=tuvar
      SigBuilderData=|
      | common.afterFinalStr = 'Extrapolate'
      | common.sampleTime = 0
      | dataSet.timeRange = [0 50]
      | dataSet.name = 'Group 1'
      | sbobj.Groups.Name = 'Group 1'
      | sbobj.Groups.Signals(1).Name = 'Yaw'
      | sbobj.Groups.Signals(1).XData = [0 2.5 10 12.5 20 27.5 30 37.5 50]
      | sbobj.Groups.Signals(1).YData = [0 0 3 3 0 -3 -3 0 0]
      | sbobj.Groups.Signals(2).Name = 'Signal 1'
      | sbobj.Groups.Signals(2).XData = [0 0.25 0.5 0.75 1 1.25 1.5 1.75 2 2.25 2.5 2.75 3 3.25 3.5 3.75 4 4.25 4.5 4.75 5 5.25 5.5 5.75 6 6.25 6.5 6.75 7 7.25 7.5 7.75 8 8.25 8.5 8.75 9 9.25 9.5 9.75 10 10.25 10.5 10.75 11 11.25 11.5 11.75 12 12.25 12.5 12.75 13 13.25 13.5 13.75 14 14.25 14.5 14.75 15 15.25 15.5 15.75 16 16.25 16.5 16.75 17 17.25 17.5 17.75 18 18.25 18.5 18.75 19 19.25 19.5 19.75 20 20.25 20.5 20.75 21 21.25 21.5 21.75 22 22.25 22.5 22.75 23 23.25 23.5 23.75 24 24.25 24.5 24.75 25 25.25 25.5 25.75 26 26.25 26.5 26.75 27 27.25 27.5 27.75 28 28.25 28.5 28.75 29 29.25 29.5 29.75 30 30.25 30.5 30.75 31 31.25 31.5 31.75 32 32.25 32.5 32.75 33 33.25 33.5 33.75 34 34.25 34.5 34.75 35 35.25 35.5 35.75 36 36.25 36.5 36.75 37 37.25 37.5 37.75 38 38.25 38.5 38.75 39 39.25 39.5 39.75 40 40.25 40.5 40.75 41 41.25 41.5 41.75 42 42.25 42.5 42.75 43 43.25 43.5 43.75 44 44.25 44.5 44.75 45 45.25 45.5 45.75 46 46.25 46.5 46.75 47 47.25 47.5 47.75 48 48.25 48.5 48.75 49 49.25 49.5 49.75 50]
      | sbobj.Groups.Signals(2).YData = [0 0.494974746831 0.7 0.494974746831 8.57252759403e-17 -0.494974746831 -0.7 -0.494974746831 0 0.494974746831 0.7 0.494974746831 ... (201 elements, 1x201)]
      | sbobj.Groups.TimeRange = [0 50]
  Yaw : Outport  Tag=STV Outport
  Signal 1 : Outport  Tag=STV Outport  Port=2
  wires:
  FromWs/1 -> Demux/1
  Demux/1 -> Yaw/1
  Demux/2 -> Signal 1/1

== system Hector/Commands/Subsystem ==
  Vx : Inport
  Vy : Inport  Port=2
  Vz : Inport  Port=3
  Yaw : Inport  Port=4
  Mux6 : Mux  Inputs=3
  Product : Product
  Product1 : Product
  Sum : Sum  Inputs=|++
  Trigonometric Function : Trigonometry
  Trigonometric Function1 : Trigonometry  Operator=cos
  V : Outport
  wires:
  Vy/1 -> Sum/2
  Vx/1 -> Product/1, Product1/1
  Product/1 -> Mux6/1
  Yaw/1 -> Trigonometric Function/1, Trigonometric Function1/1
  Sum/1 -> Mux6/2
  Trigonometric Function1/1 -> Product/2
  Product1/1 -> Sum/1
  Trigonometric Function/1 -> Product1/2
  Mux6/1 -> V/1
  Vz/1 -> Mux6/3

== system Hector/Commands/Velocity signal ==
  Demux : Demux  Tag=STV Demux  Outputs=1
      settings: DisplayOption=none
  FromWs : FromWorkspace  Tag=STV FromWs  VariableName=tuvar
      SigBuilderData=|
      | common.afterFinalStr = 'Extrapolate'
      | common.sampleTime = 0
      | dataSet.timeRange = [0 10]
      | dataSet.name = 'Group 1'
      | sbobj.Groups.Name = 'Group 1'
      | sbobj.Groups.Signals.Name = 'Signal 1'
      | sbobj.Groups.Signals.XData = [0 2 8 10]
      | sbobj.Groups.Signals.YData = [0 1 1 0]
  Signal 1 : Outport  Tag=STV Outport
  wires:
  Demux/1 -> Signal 1/1
  FromWs/1 -> Demux/1

== system Hector/Controllers/MPC Stance-leg ==
  des_state : Inport
  measBody : Inport  Port=2
  q : Inport  Port=3
  fpfv : Inport  Port=4
  Bus Selector : BusSelector  OutputSignals=rpy,x,y,z,wx,wy,wz,vx,vy,vz
  MPC controller : MATLABFcn  MATLABFcn=LocomotionMPC_qpoases  OutputDimensions=[12 1]  Output1D=off
  Mapping : MATLABFcn  MATLABFcn=JacobianMapping  OutputDimensions=[10 1]  Output1D=off
  Mux : Mux
  Mux1 : Mux  Inputs=10
  Mux2 : Mux  Inputs=3
  Rate Transition : RateTransition  OutPortSampleTime=dt_MPC/5
  Rate Transition1 : RateTransition  OutPortSampleTime=0.001
  To Workspace : ToWorkspace  VariableName=MPCForce  SampleTime=-1
      settings: Save2DSignal=2-D array (concatenate along first dimension)
  Transpose : Math  Operator=transpose
  tau : Outport
  wires:
  measBody/1 -> Bus Selector/1
  des_state/1 -> Mux/1
  Mux/1 -> Rate Transition/1
  Bus Selector/1 -> Mux1/1  "<rpy>"
  Bus Selector/2 -> Mux1/2  "<x>"
  Bus Selector/3 -> Mux1/3  "<y>"
  Bus Selector/4 -> Mux1/4  "<z>"
  Bus Selector/5 -> Mux1/5  "<wx>"
  Bus Selector/6 -> Mux1/6  "<wy>"
  Bus Selector/7 -> Mux1/7  "<wz>"
  Bus Selector/8 -> Mux1/8  "<vx>"
  Bus Selector/9 -> Mux1/9  "<vy>"
  Bus Selector/10 -> Mux1/10  "<vz>"
  q/1 -> Mux2/2, Mux/3
  Rate Transition/1 -> MPC controller/1
  MPC controller/1 -> Mux2/3, Transpose/1  "F_MPC"
  Mapping/1 -> tau/1
  fpfv/1 -> Mux/4
  Rate Transition1/1 -> To Workspace/1
  Transpose/1 -> Rate Transition1/1
  Mux2/1 -> Mapping/1
  Mux1/1 -> Mux2/1, Mux/2

== system Hector/Controllers/Meas Conn ==
  In1 : Inport
  In2 : Inport  Port=2
  Bus Selector : BusSelector  OutputSignals=hip_yaw_angle,hip_roll_angle,hip_pitch_angle,knee_angle,ankle_angle  OutputAsBus=on
  Bus Selector1 : BusSelector  OutputSignals=hip_yaw_angle,hip_roll_angle,hip_pitch_angle,knee_angle,ankle_angle  OutputAsBus=on
  Bus Selector2 : BusSelector  OutputSignals=hip_location_r
  Bus Selector3 : BusSelector  OutputSignals=hip_location_l
  Bus Selector5 : BusSelector  OutputSignals=hip_yaw_speed,hip_roll_speed,hip_pitch_speed,knee_speed,ankle_speed  OutputAsBus=on
  Bus Selector6 : BusSelector  OutputSignals=hip_yaw_speed,hip_roll_speed,hip_pitch_speed,knee_speed,ankle_speed  OutputAsBus=on
  Bus Selector7 : BusSelector  OutputSignals=foot_pos_vel_r
  Bus Selector8 : BusSelector  OutputSignals=foot_pos_vel_l
  Mux{,1..3} (4 alike) : Mux  Inputs=2
  Out1 : Outport
  qd : Outport  Port=2
  fpfv : Outport  Port=3
  q : Outport  Port=4
  wires:
  In2/1 -> Bus Selector8/1, Bus Selector6/1, Bus Selector3/1, Bus Selector1/1
  Bus Selector8/1 -> Mux3/2  "<foot_pos_vel_l>"
  Bus Selector5/1 -> Mux2/1  "qd_r"
  Bus Selector2/1 -> Mux1/1  "<hip_location_r>"
  Bus Selector3/1 -> Mux1/2  "<hip_location_l>"
  Mux/1 -> q/1  "q"
  In1/1 -> Bus Selector7/1, Bus Selector5/1, Bus Selector2/1, Bus Selector/1
  Bus Selector/1 -> Mux/1  "q_r"
  Bus Selector1/1 -> Mux/2  "q_l"
  Mux2/1 -> qd/1  "qd"
  Bus Selector6/1 -> Mux2/2  "qd_l"
  Bus Selector7/1 -> Mux3/1  "<foot_pos_vel_r>"
  Mux3/1 -> fpfv/1  "fpfv"
  Mux1/1 -> Out1/1

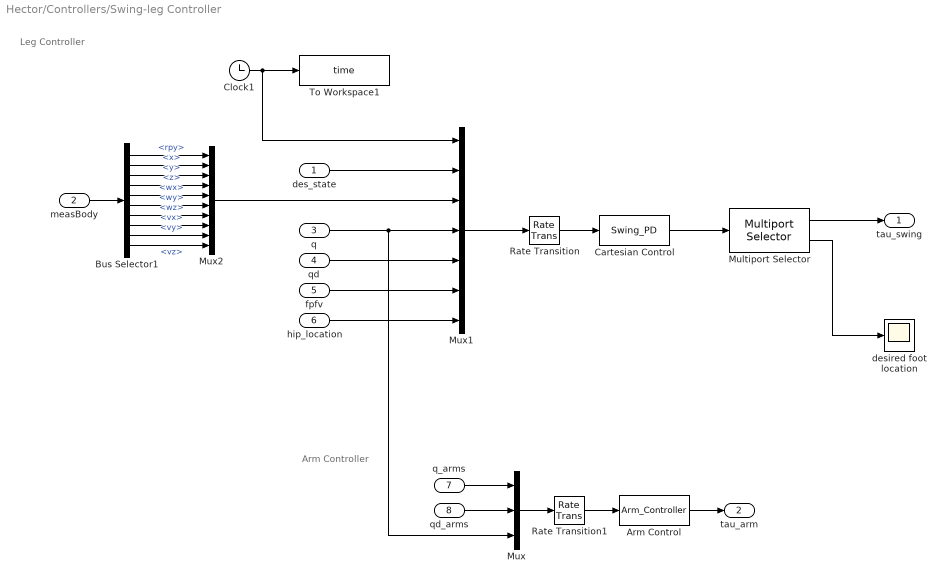
== system Hector/Controllers/Swing-leg Controller  ==
  note: Arm Controller
  note: Leg Controller
  des_state : Inport
  measBody : Inport  Port=2
  q : Inport  Port=3
  qd : Inport  Port=4
  fpfv : Inport  Port=5
  hip_location : Inport  Port=6
  q_arms : Inport  Port=7
  qd_arms : Inport  Port=8
  Arm Control : MATLABFcn  MATLABFcn=Arm_Controller  Output1D=off
  Bus Selector1 : BusSelector  OutputSignals=rpy,x,y,z,wx,wy,wz,vx,vy,vz
  Cartesian Control : MATLABFcn  MATLABFcn=Swing_PD  Output1D=off
  Clock1 : Clock
  Multiport Selector : dspindex/Multiport Selector  rowsOrCols=Rows  idxCellArray={ 1:10, 11:20}  idxErrMode=Clip Index
  Mux : Mux  Inputs=3
  Mux1 : Mux  Inputs=7
  Mux2 : Mux  Inputs=10
  Rate Transition : RateTransition  OutPortSampleTime=0.001
  Rate Transition1 : RateTransition  OutPortSampleTime=0.001
  To Workspace1 : ToWorkspace  VariableName=time  SampleTime=-1
  desired foot location : Scope
  tau_swing : Outport
  tau_arm : Outport  Port=2
  wires:
  Rate Transition/1 -> Cartesian Control/1
  Cartesian Control/1 -> Multiport Selector/1
  Multiport Selector/1 -> tau_swing/1
  Multiport Selector/2 -> desired foot location/1
  Mux2/1 -> Mux1/3
  Bus Selector1/4 -> Mux2/4  "<z>"
  Bus Selector1/1 -> Mux2/1  "<rpy>"
  Bus Selector1/7 -> Mux2/7  "<wz>"
  Bus Selector1/5 -> Mux2/5  "<wx>"
  Bus Selector1/8 -> Mux2/8  "<vx>"
  Bus Selector1/9 -> Mux2/9  "<vy>"
  qd/1 -> Mux1/5
  des_state/1 -> Mux1/2
  hip_location/1 -> Mux1/7
  Mux1/1 -> Rate Transition/1
  fpfv/1 -> Mux1/6
  measBody/1 -> Bus Selector1/1
  Bus Selector1/6 -> Mux2/6  "<wy>"
  q/1 -> Mux/3, Mux1/4
  Bus Selector1/2 -> Mux2/2  "<x>"
  Bus Selector1/10 -> Mux2/10  "<vz>"
  Bus Selector1/3 -> Mux2/3  "<y>"
  Clock1/1 -> Mux1/1, To Workspace1/1
  Rate Transition1/1 -> Arm Control/1
  Arm Control/1 -> tau_arm/1
  Mux/1 -> Rate Transition1/1
  q_arms/1 -> Mux/1
  qd_arms/1 -> Mux/2
